simulink model "car_simulation"  (R2022a)
settings: Solver=VariableStepAuto  StartTime=0.0  StopTime=8  RelTol=1e-3
settings Model: Creator=Rehan Binu Kuruvilla  LastModifiedBy=Rehan Binu Kuruvilla

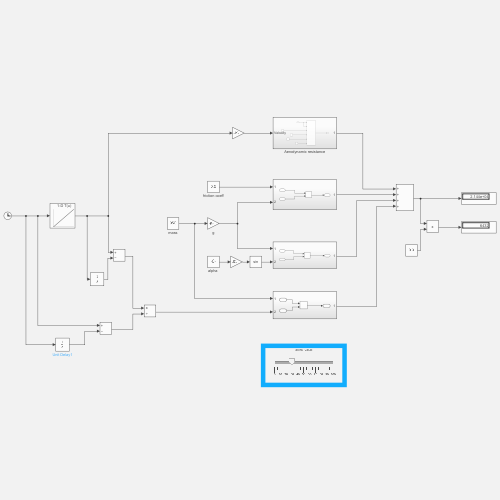
[thumbnail: Simulink's stored preview of the top-level diagram]
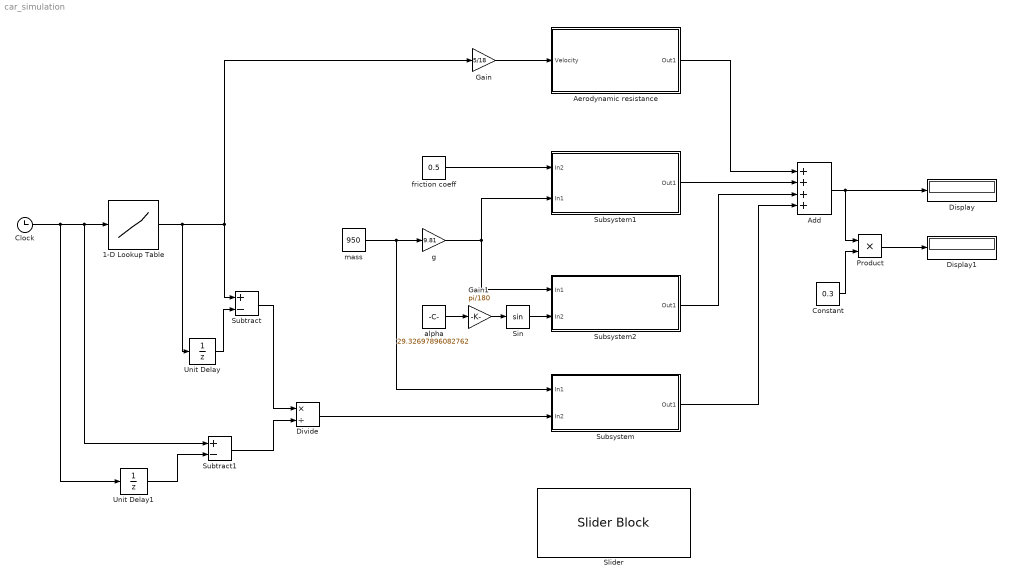
== system car_simulation ==
  1-D Lookup Table : Lookup_n-D  NumberOfTableDimensions=1  BreakpointsForDimension1=[0 8]  Table=[0 100]  InternalRulePriority=Speed  RndMeth=Simplest
  Add : Sum  Inputs=++++
  Aerodynamic resistance : Subsystem
  Clock : Clock
  Constant : Constant  Value=0.3
  Display : Display
  Display1 : Display
  Divide : Product  Inputs=*/
  Gain : Gain  Gain=5/18
  Gain1 : Gain  Gain=pi/180
  Product : Product
  Sin : Trigonometry
  Slider : SliderBlock
  Subsystem : Subsystem
  Subsystem1 : Subsystem
  Subsystem2 : Subsystem
  Subtract : Sum  Inputs=+-
  Subtract1 : Sum  Inputs=+-
  Unit Delay : UnitDelay  SampleTime=-1  HasFrameUpgradeWarning=on
  Unit Delay1 : UnitDelay  SampleTime=-1  HasFrameUpgradeWarning=on
  "alpha " : Constant  Value=29.32697896082762
  friction coeff : Constant  Value=0.5
  g : Gain  Gain=9.81
  mass : Constant  Value=950
  wires:
  Clock/1 -> Unit Delay1/1, Subtract1/1, 1-D Lookup Table/1
  Gain/1 -> Aerodynamic resistance/1(Velocity)
  mass/1 -> Subsystem/1(In1), g/1
  g/1 -> Subsystem1/2(In1), Subsystem2/1(In1)
  "alpha "/1 -> Gain1/1
  Sin/1 -> Subsystem2/2(In2)
  friction coeff/1 -> Subsystem1/1(In2)
  Aerodynamic resistance/1(Out1) -> Add/1
  Subsystem1/1(Out1) -> Add/2
  Subsystem2/1(Out1) -> Add/3
  Add/1 -> Display/1, Product/1
  Gain1/1 -> Sin/1
  1-D Lookup Table/1 -> Gain/1, Subtract/1, Unit Delay/1
  Subsystem/1(Out1) -> Add/4
  Constant/1 -> Product/2
  Product/1 -> Display1/1
  Unit Delay/1 -> Subtract/2
  Subtract/1 -> Divide/1
  Unit Delay1/1 -> Subtract1/2
  Subtract1/1 -> Divide/2
  Divide/1 -> Subsystem/2(In2)

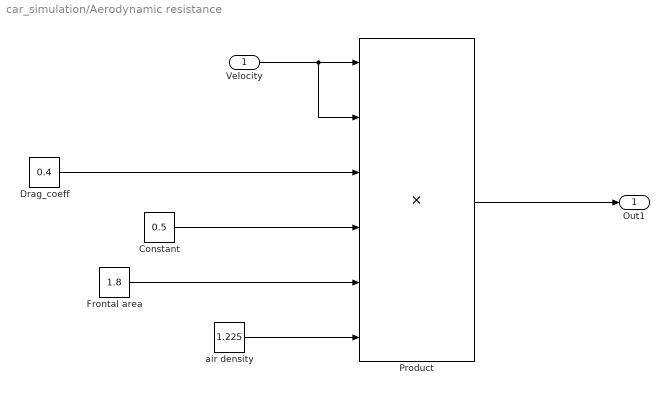
== system car_simulation/Aerodynamic resistance ==
  Velocity : Inport
  Constant : Constant  Value=0.5
  Drag_coeff : Constant  Value=0.4
  Frontal area : Constant  Value=1.8
  Product : Product  Inputs=6
  air density : Constant  Value=1.225
  Out1 : Outport
  wires:
  Velocity/1 -> Product/2, Product/1
  air density/1 -> Product/6
  Drag_coeff/1 -> Product/3
  Frontal area/1 -> Product/5
  Constant/1 -> Product/4
  Product/1 -> Out1/1

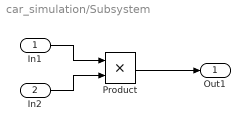
== system car_simulation/Subsystem ==
  In1 : Inport
  In2 : Inport  Port=2
  Product : Product
  Out1 : Outport
  wires:
  In1/1 -> Product/1
  In2/1 -> Product/2
  Product/1 -> Out1/1

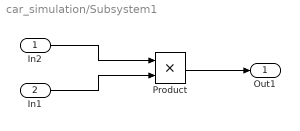
== system car_simulation/Subsystem1 ==
  In2 : Inport
  In1 : Inport  Port=2
  Product : Product
  Out1 : Outport
  wires:
  In1/1 -> Product/2
  In2/1 -> Product/1
  Product/1 -> Out1/1

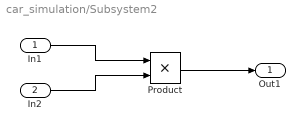
== system car_simulation/Subsystem2 ==
  In1 : Inport
  In2 : Inport  Port=2
  Product : Product
  Out1 : Outport
  wires:
  In1/1 -> Product/1
  In2/1 -> Product/2
  Product/1 -> Out1/1
